simulink model "simu3_SISO"  (R2015b)
settings: Solver=ode45  StartTime=0.0  StopTime=100  RelTol=1e-3
undefined symbols (not defined in the file or in its folder): a0, a1, am, b0, bm, F, g, kp
settings Model: Creator=Wissale !  LastModifiedBy=Kais_Mesfioui
settings DataIOCC: SaveFormat=Array
settings DebuggingCC: SolverPrmCheckMsg=warning
settings HardwareCC: ProdBitPerPointer=32  ProdLargestAtomicFloat=None  ProdIntDivRoundTo=Undefined  ProdEndianess=Unspecified  ProdWordSize=32  ProdHWDeviceType=32-bit Generic
settings GRTTargetCC: GeneratePreprocessorConditionals=Disable all
settings ConfigComp: CovModelRefEnable=Off  CovSFcnEnable=off

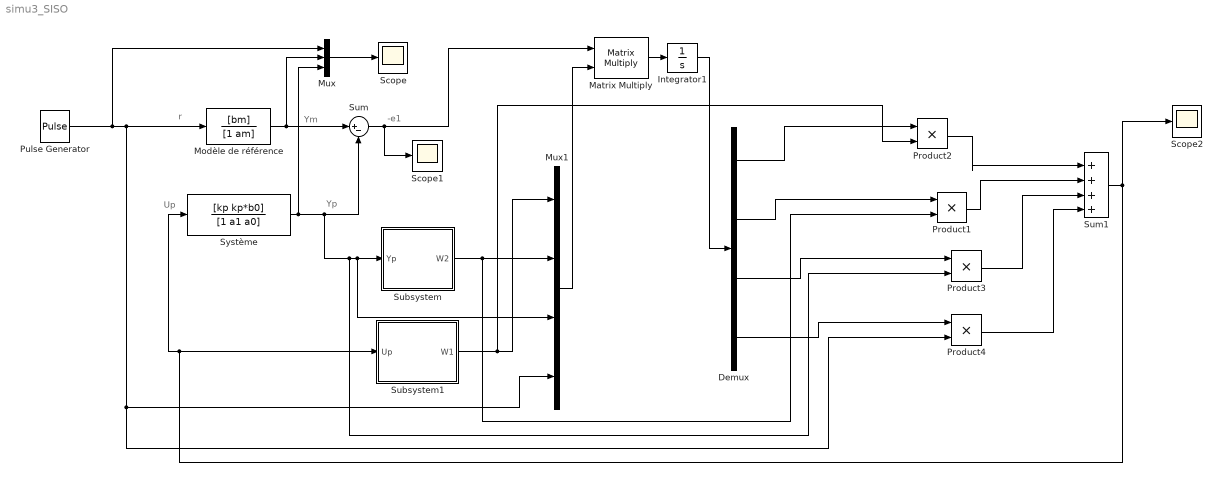
== system simu3_SISO ==
  note: -e1
  note: r
  note: Up
  note: Ym
  note: Yp
  Demux : Demux
  Integrator1 : Integrator  InitialCondition=0.01
  Matrix Multiply : Product  Multiplication=Matrix(*)
  Modèle de référence : TransferFcn  Numerator=[bm]  Denominator=[1 am]
  Mux : Mux  Inputs=3
  Mux1 : Mux
  Product{1..4} (4 alike) : Product
  Pulse Generator : DiscretePulseGenerator  PulseType=Time based  Period=20  PulseWidth=50
  Scope : Scope
  Scope1 : Scope
  Scope2 : Scope
  Subsystem : Subsystem
  Subsystem1 : Subsystem
  Sum : Sum  Inputs=|+-
  Sum1 : Sum  Inputs=|++++
  Système : TransferFcn  Numerator=[kp kp*b0]  Denominator=[1 a1 a0]
  wires:
  Pulse Generator/1 -> Mux/1, Product4/2, Mux1/4, Modèle de référence/1
  Système/1 -> Product3/2, Mux1/3, Subsystem/1(Yp), Sum/2, Mux/3
  Subsystem1/1(W1) -> Product2/2, Mux1/1
  Subsystem/1(W2) -> Product1/2, Mux1/2
  Mux1/1 -> Matrix Multiply/2
  Sum/1 -> Scope1/1, Matrix Multiply/1
  Matrix Multiply/1 -> Integrator1/1
  Integrator1/1 -> Demux/1
  Demux/1 -> Product2/1
  Product2/1 -> Sum1/1
  Demux/2 -> Product1/1
  Product1/1 -> Sum1/2
  Demux/3 -> Product3/1
  Product3/1 -> Sum1/3
  Demux/4 -> Product4/1
  Product4/1 -> Sum1/4
  Sum1/1 -> Système/1, Subsystem1/1(Up), Scope2/1
  Modèle de référence/1 -> Mux/2, Sum/1
  Mux/1 -> Scope/1

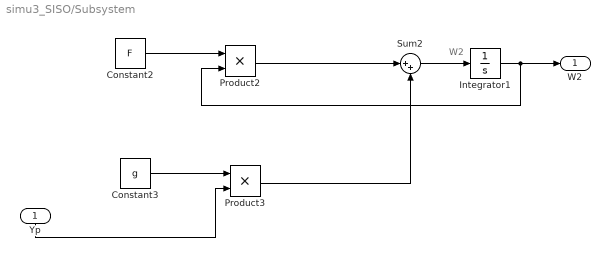
== system simu3_SISO/Subsystem ==
  note: W2
  Yp : Inport
  Constant2 : Constant  Value=F
  Constant3 : Constant  Value=g
  Integrator1 : Integrator
  Product2 : Product
  Product3 : Product
  Sum2 : Sum  Inputs=|++
  W2 : Outport
  wires:
  Yp/1 -> Product3/2
  Sum2/1 -> Integrator1/1
  Constant2/1 -> Product2/1
  Constant3/1 -> Product3/1
  Product3/1 -> Sum2/2
  Integrator1/1 -> Product2/2, W2/1
  Product2/1 -> Sum2/1

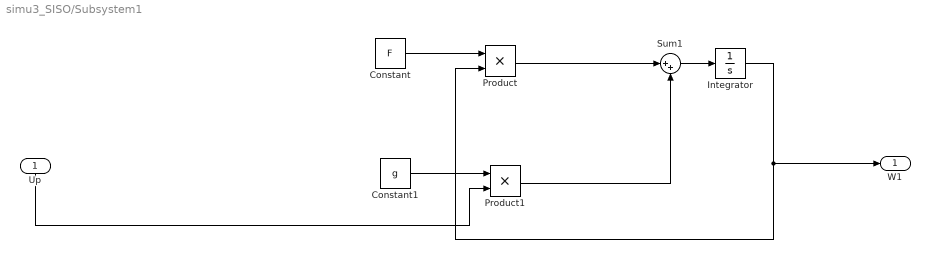
== system simu3_SISO/Subsystem1 ==
  Up : Inport
  Constant : Constant  Value=F
  Constant1 : Constant  Value=g
  Integrator : Integrator
  Product : Product
  Product1 : Product
  Sum1 : Sum  Inputs=|++
  W1 : Outport
  wires:
  Product/1 -> Sum1/1
  Constant1/1 -> Product1/1
  Product1/1 -> Sum1/2
  Up/1 -> Product1/2
  Constant/1 -> Product/1
  Sum1/1 -> Integrator/1
  Integrator/1 -> Product/2, W1/1
